simulink model "fcn"  (R2019b)
settings: Solver=VariableStepAuto  StartTime=0.0  StopTime=5  RelTol=1e-2
settings Model: Creator=fang  LastModifiedBy=fang

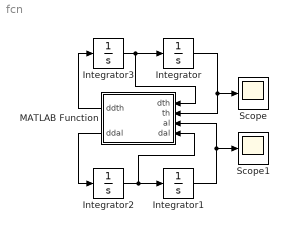
== system fcn ==
  Integrator : Integrator
  Integrator1 : Integrator  InitialCondition=pi/60
  Integrator2 : Integrator
  Integrator3 : Integrator
  MATLAB Function : MATLAB Function  TreatAsAtomicUnit=on
  Scope : Scope
  Scope1 : Scope
  wires:
  Integrator2/1 -> MATLAB Function/4(dal), Integrator1/1
  Integrator3/1 -> MATLAB Function/1(dth), Integrator/1
  MATLAB Function/1(ddth) -> Integrator3/1
  MATLAB Function/2(ddal) -> Integrator2/1
  Integrator/1 -> Scope/1, MATLAB Function/2(th)
  Integrator1/1 -> MATLAB Function/3(al), Scope1/1

== matlab function fcn/MATLAB Function ==
  data: dth input; th input; al input; dal input; ddth output; ddal output
function [ddth, ddal] = fcn(dth,th,al,dal)
% inputs: th: theta, al: alpha, dth: d(theta)/dt, dal: d(alpha)/dt
% outputs: ddth: d^2(theta)/dt^2, ddal: d^2(alpha)/dt^2
k_al = 0.0005; k_th = 0.0001;

D = [-0.0031*cos(al)^2+0.011, 0.0043*cos(al); 0.0043*cos(al), 0.0043];

C = [0.0061*cos(al)*dal*sin(al), -0.0043*sin(al)*dal; -0.0031*cos(al)*dth*sin(al), 0];

g = [0; 0.1939*sin(al)];

M = [-0.0024*dth-k_th*sign(dth); -0.0024*dal-k_al*sign(dal)];

outputs = D\(M-g-C*[dth; dal]);

ddth = outputs(1); ddal = outputs(2);
